simulink model "mask_system"  (R2022b)
settings: Solver=VariableStepAuto  StartTime=0.0  StopTime=10.0  RelTol=1e-3
settings Model: Creator=Dell  LastModifiedBy=Dell

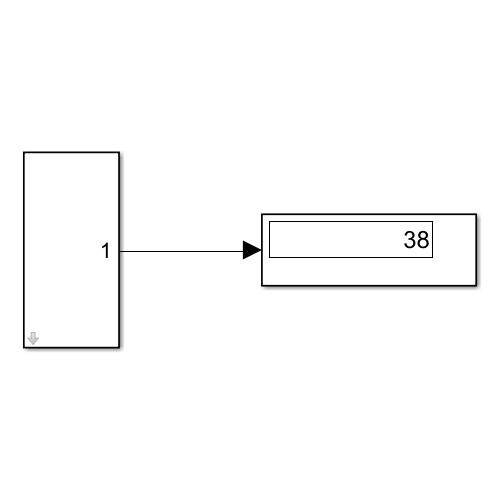
[thumbnail: Simulink's stored preview of the top-level diagram]
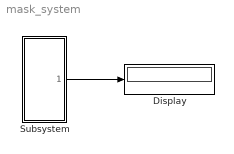
== system mask_system ==
  Display : Display
  Subsystem : Subsystem  mask{const=18, const1=20, data=int16}
      mask prompts: const "p1"; const1 "p2"; data "type"
  wires:
  Subsystem/1(Outport) -> Display/1

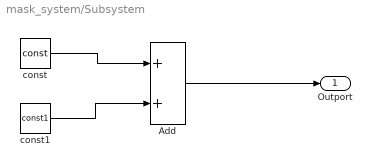
== system mask_system/Subsystem ==
  Add : Sum
  const : Constant  Value=const
  const1 : Constant  Value=const1
  Outport : Outport
  wires:
  Add/1 -> Outport/1
  const/1 -> Add/1
  const1/1 -> Add/2
